simulink model "FacundoADProject2017a"  (R2017a)
settings: Solver=VariableStepAuto  StartTime=0.0  StopTime=5930  RelTol=1e-3
libraries: simulink x4, vrlib x3
settings Model: Creator=izacu  LastModifiedBy=izacu
settings DataIOCC: ReturnWorkspaceOutputs=on
settings DebuggingCC: UnconnectedInputMsg=none  UnconnectedOutputMsg=none  UnconnectedLineMsg=none  SFMachineParentedDataDiag=error
settings ModelReferenceCC: EnableRefExpFcnMdlSchedulingChecks=off
settings SFSimCC: SimUseLocalCustomCode=on
settings RTWCC: RTWUseLocalCustomCode=on

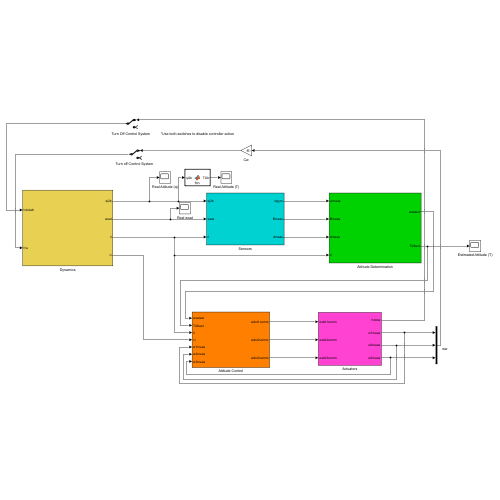
[thumbnail: Simulink's stored preview of the top-level diagram]
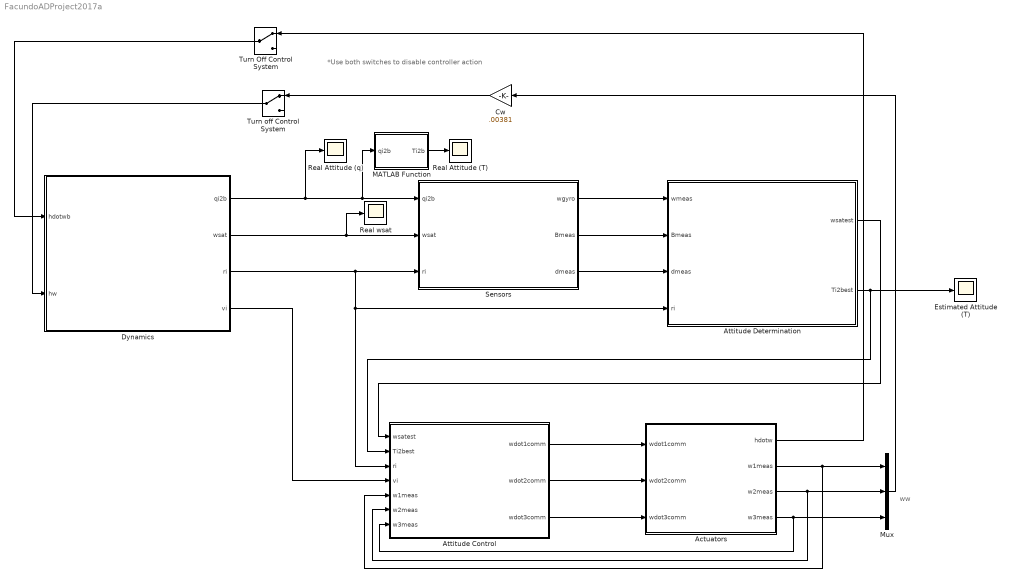
== system FacundoADProject2017a ==
  note: *Use both switches to disable controller action
  note: ww
  Actuators : Subsystem
  Attitude Control : Subsystem
  Attitude Determination : Subsystem
  Cw : Gain  Gain=.00381
  Dynamics : Subsystem
  Estimated Attitude (T) : Scope
  MATLAB Function : MATLAB Function  TreatAsAtomicUnit=on
  Mux : Mux  Inputs=3
  Real Attitude (T) : Scope
  Real Attitude (q) : Scope
  Real wsat : Scope
  Sensors : Subsystem
  Turn Off Control System : ManualSwitch
  Turn off Control System : ManualSwitch
  wires:
  Actuators/2(w1meas) -> Attitude Control/5(w1meas), Mux/1
  Actuators/3(w2meas) -> Attitude Control/6(w2meas), Mux/2
  Actuators/4(w3meas) -> Attitude Control/7(w3meas), Mux/3
  Dynamics/1(qi2b) -> Real Attitude (q)/1, MATLAB Function/1(qi2b), Sensors/1(qi2b)
  Sensors/1(wgyro) -> Attitude Determination/1(wmeas)
  Sensors/2(Bmeas) -> Attitude Determination/2(Bmeas)
  Sensors/3(dmeas) -> Attitude Determination/3(dmeas)
  Dynamics/3(ri) -> Attitude Control/3(ri), Attitude Determination/4(ri), Sensors/3(ri)
  Dynamics/2(wsat) -> Real wsat/1, Sensors/2(wsat)
  Attitude Control/1(wdot1comm) -> Actuators/1(wdot1comm)
  Attitude Control/2(wdot2comm) -> Actuators/2(wdot2comm)
  Attitude Control/3(wdot3comm) -> Actuators/3(wdot3comm)
  Dynamics/4(vi) -> Attitude Control/4(vi)
  Attitude Determination/1(wsatest) -> Attitude Control/1(wsatest)
  Attitude Determination/2(Ti2best) -> Attitude Control/2(Ti2best), Estimated Attitude (T)/1
  Mux/1 -> Cw/1
  MATLAB Function/1(Ti2b) -> Real Attitude (T)/1
  Turn off Control System/1 -> Dynamics/2(hw)
  Cw/1 -> Turn off Control System/1
  Turn Off Control System/1 -> Dynamics/1(hdotwb)
  Actuators/1(hdotw) -> Turn Off Control System/1

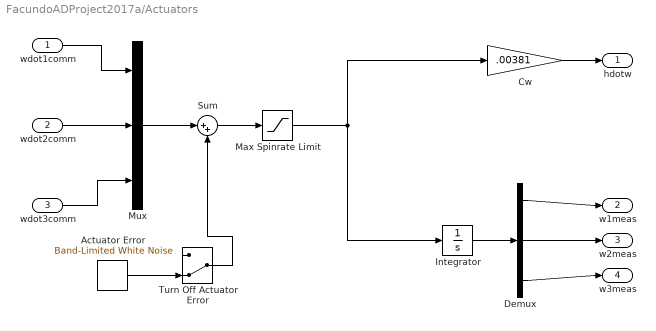
== system FacundoADProject2017a/Actuators ==
  wdot1comm : Inport
  wdot2comm : Inport  Port=2
  wdot3comm : Inport  Port=3
  Actuator Error : simulink/Sources/Band-Limited White Noise  Cov=2 * [1;1;1]  Ts=0.1  seed=[23341]
  Cw : Gain  Gain=.00381
  Demux : Demux  Outputs=3
  Integrator : Integrator  InitialCondition=[0;0;0]
  Max Spinrate Limit : Saturate  UpperLimit=262*[1;1;1]  LowerLimit=-262*[1;1;1]
  Mux : Mux  Inputs=3
  Sum : Sum  Inputs=|++
  Turn Off Actuator Error : ManualSwitch  CurrentSetting=0
  hdotw : Outport
  w1meas : Outport  Port=2
  w2meas : Outport  Port=3
  w3meas : Outport  Port=4
  wires:
  wdot1comm/1 -> Mux/1
  wdot2comm/1 -> Mux/2
  wdot3comm/1 -> Mux/3
  Mux/1 -> Sum/1
  Sum/1 -> Max Spinrate Limit/1
  Integrator/1 -> Demux/1
  Demux/1 -> w1meas/1
  Demux/2 -> w2meas/1
  Demux/3 -> w3meas/1
  Cw/1 -> hdotw/1
  Actuator Error/1 -> Turn Off Actuator Error/2
  Turn Off Actuator Error/1 -> Sum/2
  Max Spinrate Limit/1 -> Cw/1, Integrator/1

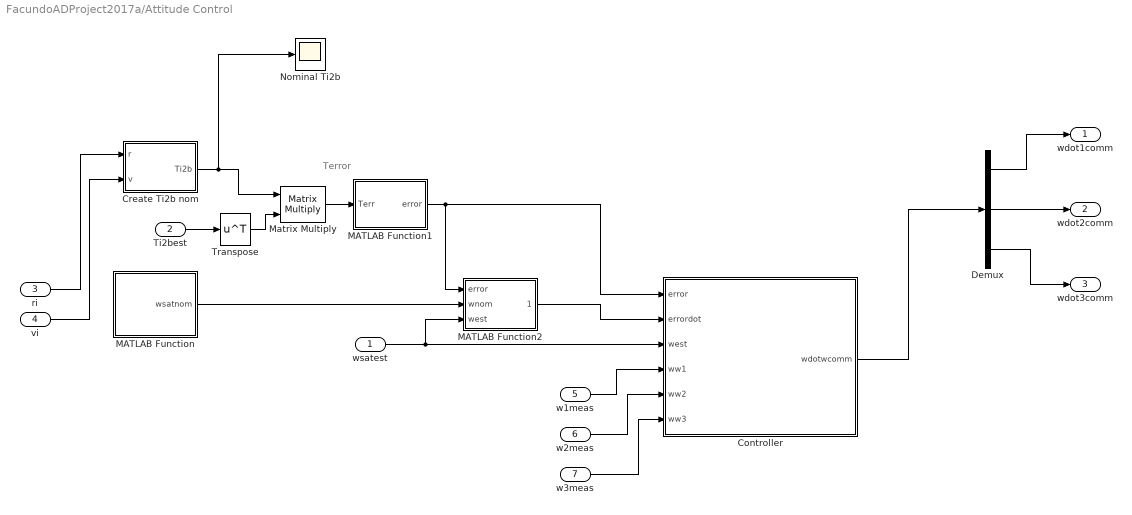
== system FacundoADProject2017a/Attitude Control ==
  note: Terror
  wsatest : Inport
  Ti2best : Inport  Port=2
  ri : Inport  Port=3
  vi : Inport  Port=4
  w1meas : Inport  Port=5
  w2meas : Inport  Port=6
  w3meas : Inport  Port=7
  Controller : MATLAB Function  TreatAsAtomicUnit=on
  Create Ti2b nom : MATLAB Function  TreatAsAtomicUnit=on
  Demux : Demux  Outputs=3
  MATLAB Function : MATLAB Function  TreatAsAtomicUnit=on
  MATLAB Function1 : MATLAB Function  TreatAsAtomicUnit=on
  MATLAB Function2 : MATLAB Function  TreatAsAtomicUnit=on
  Matrix Multiply : Product  Multiplication=Matrix(*)
  Nominal Ti2b : Scope
  Transpose : Math  Operator=transpose  SaturateOnIntegerOverflow=on
  wdot1comm : Outport
  wdot2comm : Outport  Port=2
  wdot3comm : Outport  Port=3
  wires:
  Demux/1 -> wdot1comm/1
  Demux/2 -> wdot2comm/1
  Demux/3 -> wdot3comm/1
  ri/1 -> Create Ti2b nom/1(r)
  vi/1 -> Create Ti2b nom/2(v)
  Create Ti2b nom/1(Ti2b) -> Nominal Ti2b/1, Matrix Multiply/1
  Matrix Multiply/1 -> MATLAB Function1/1(Terr)
  MATLAB Function1/1(error) -> Controller/1(error), MATLAB Function2/1(error)
  MATLAB Function/1(wsatnom) -> MATLAB Function2/2(wnom)
  wsatest/1 -> Controller/3(west), MATLAB Function2/3(west)
  Controller/1(wdotwcomm) -> Demux/1
  w1meas/1 -> Controller/4(ww1)
  w2meas/1 -> Controller/5(ww2)
  w3meas/1 -> Controller/6(ww3)
  MATLAB Function2/1(errordot) -> Controller/2(errordot)
  Ti2best/1 -> Transpose/1
  Transpose/1 -> Matrix Multiply/2

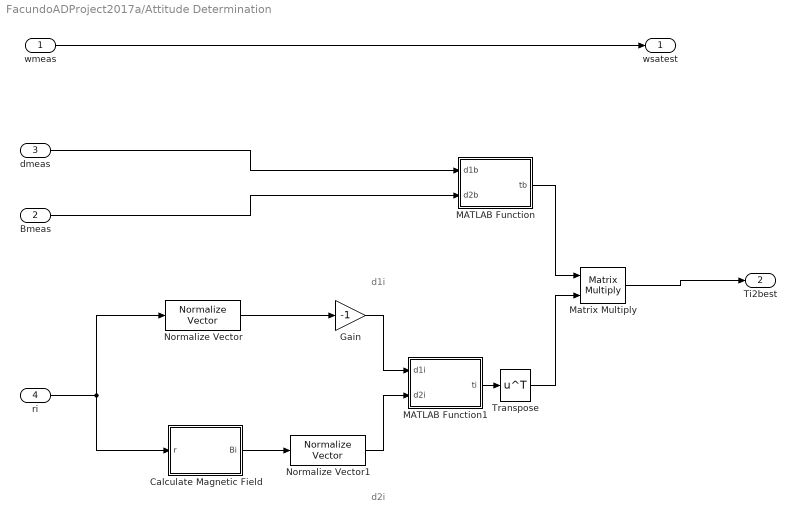
== system FacundoADProject2017a/Attitude Determination ==
  note: d2i
  note: d1i
  wmeas : Inport
  Bmeas : Inport  Port=2
  dmeas : Inport  Port=3
  ri : Inport  Port=4
  Calculate Magnetic Field : MATLAB Function  TreatAsAtomicUnit=on
  Gain : Gain  Gain=-1
  MATLAB Function : MATLAB Function  TreatAsAtomicUnit=on
  MATLAB Function1 : MATLAB Function  TreatAsAtomicUnit=on
  Matrix Multiply : Product  Multiplication=Matrix(*)
  Normalize Vector : vrlib/Utilities/Normalize Vector  maxzero=0
  Normalize Vector1 : vrlib/Utilities/Normalize Vector  maxzero=0
  Transpose : Math  Operator=transpose  SaturateOnIntegerOverflow=on
  wsatest : Outport
  Ti2best : Outport  Port=2
  wires:
  wmeas/1 -> wsatest/1
  ri/1 -> Normalize Vector/1, Calculate Magnetic Field/1(r)
  Calculate Magnetic Field/1(Bi) -> Normalize Vector1/1
  Normalize Vector/1 -> Gain/1
  dmeas/1 -> MATLAB Function/1(d1b)
  Bmeas/1 -> MATLAB Function/2(d2b)
  Gain/1 -> MATLAB Function1/1(d1i)
  Normalize Vector1/1 -> MATLAB Function1/2(d2i)
  MATLAB Function1/1(ti) -> Transpose/1
  MATLAB Function/1(tb) -> Matrix Multiply/1
  Transpose/1 -> Matrix Multiply/2
  Matrix Multiply/1 -> Ti2best/1

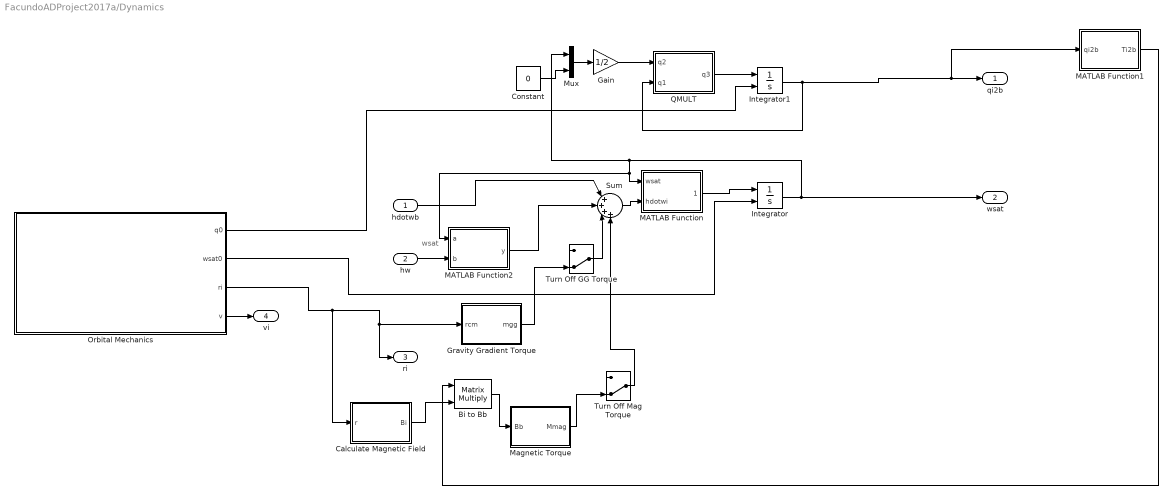
== system FacundoADProject2017a/Dynamics ==
  note: wsat
  hdotwb : Inport
  hw : Inport  Port=2
  Bi to Bb : Product  Multiplication=Matrix(*)
  Calculate Magnetic Field : MATLAB Function  TreatAsAtomicUnit=on
  Constant : Constant  Value=0
  Gain : Gain  Gain=1/2
  Gravity Gradient Torque : MATLAB Function  TreatAsAtomicUnit=on
  Integrator : Integrator  InitialConditionSource=external
  Integrator1 : Integrator  InitialConditionSource=external
  MATLAB Function : MATLAB Function  TreatAsAtomicUnit=on
  MATLAB Function1 : MATLAB Function  TreatAsAtomicUnit=on
  MATLAB Function2 : MATLAB Function  TreatAsAtomicUnit=on
  Magnetic Torque : MATLAB Function  TreatAsAtomicUnit=on
  Mux : Mux  Inputs=2
  Orbital Mechanics : Subsystem
  QMULT : MATLAB Function  TreatAsAtomicUnit=on
  Sum : Sum  Inputs=|++++
  Turn Off GG Torque : ManualSwitch  CurrentSetting=0
  Turn Off Mag Torque : ManualSwitch  CurrentSetting=0
  qi2b : Outport
  wsat : Outport  Port=2
  ri : Outport  Port=3
  vi : Outport  Port=4
  wires:
  hw/1 -> MATLAB Function2/2(b)
  hdotwb/1 -> Sum/1
  Sum/1 -> MATLAB Function/2(hdotwi)
  MATLAB Function/1(wdotsat) -> Integrator/1
  Integrator/1 -> wsat/1, Mux/1, MATLAB Function2/1(a), MATLAB Function/1(wsat)
  Orbital Mechanics/3(ri) -> Gravity Gradient Torque/1(rcm), ri/1, Calculate Magnetic Field/1(r)
  Orbital Mechanics/4(v) -> vi/1
  Orbital Mechanics/2(wsat0) -> Integrator/2
  Integrator1/1 -> QMULT/2(q1), MATLAB Function1/1(qi2b), qi2b/1
  QMULT/1(q3) -> Integrator1/1
  Mux/1 -> Gain/1
  Constant/1 -> Mux/2
  Orbital Mechanics/1(q0) -> Integrator1/2
  Gain/1 -> QMULT/1(q2)
  Calculate Magnetic Field/1(Bi) -> Bi to Bb/2
  MATLAB Function1/1(Ti2b) -> Bi to Bb/1
  Bi to Bb/1 -> Magnetic Torque/1(Bb)
  Magnetic Torque/1(Mmag) -> Turn Off Mag Torque/2
  Turn Off Mag Torque/1 -> Sum/4
  Gravity Gradient Torque/1(mgg) -> Turn Off GG Torque/2
  Turn Off GG Torque/1 -> Sum/3
  MATLAB Function2/1(y) -> Sum/2

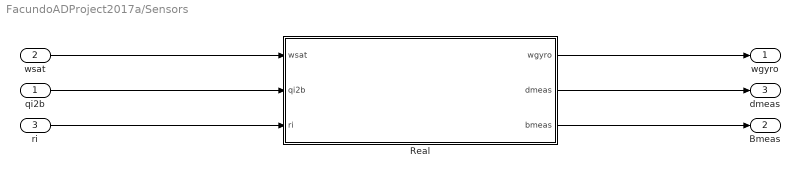
== system FacundoADProject2017a/Sensors ==
  qi2b : Inport
  wsat : Inport  Port=2
  ri : Inport  Port=3
  Real : Subsystem
  wgyro : Outport
  Bmeas : Outport  Port=2
  dmeas : Outport  Port=3
  wires:
  wsat/1 -> Real/1(wsat)
  qi2b/1 -> Real/2(qi2b)
  ri/1 -> Real/3(ri)
  Real/1(wgyro) -> wgyro/1
  Real/2(dmeas) -> dmeas/1
  Real/3(bmeas) -> Bmeas/1

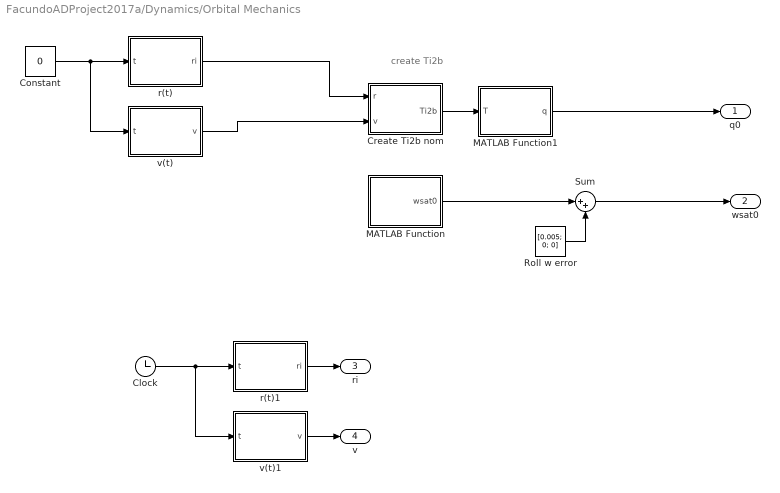
== system FacundoADProject2017a/Dynamics/Orbital Mechanics ==
  note: create Ti2b
  Clock : Clock
  Constant : Constant  Value=0
  Create Ti2b nom : MATLAB Function  TreatAsAtomicUnit=on
  MATLAB Function : MATLAB Function  TreatAsAtomicUnit=on
  MATLAB Function1 : MATLAB Function  TreatAsAtomicUnit=on
  Roll w error : Constant  Value=[0.005; 0; 0]
  Sum : Sum  Inputs=|++
  r(t) : MATLAB Function  TreatAsAtomicUnit=on
  r(t)1 : MATLAB Function  TreatAsAtomicUnit=on
  v(t) : MATLAB Function  TreatAsAtomicUnit=on
  v(t)1 : MATLAB Function  TreatAsAtomicUnit=on
  q0 : Outport
  wsat0 : Outport  Port=2
  ri : Outport  Port=3
  v : Outport  Port=4
  wires:
  Constant/1 -> v(t)/1(t), r(t)/1(t)
  v(t)/1(v) -> Create Ti2b nom/2(v)
  r(t)/1(ri) -> Create Ti2b nom/1(r)
  Roll w error/1 -> Sum/2
  MATLAB Function/1(wsat0) -> Sum/1
  Sum/1 -> wsat0/1
  Create Ti2b nom/1(Ti2b) -> MATLAB Function1/1(T)
  MATLAB Function1/1(q) -> q0/1
  Clock/1 -> v(t)1/1(t), r(t)1/1(t)
  r(t)1/1(ri) -> ri/1
  v(t)1/1(v) -> v/1

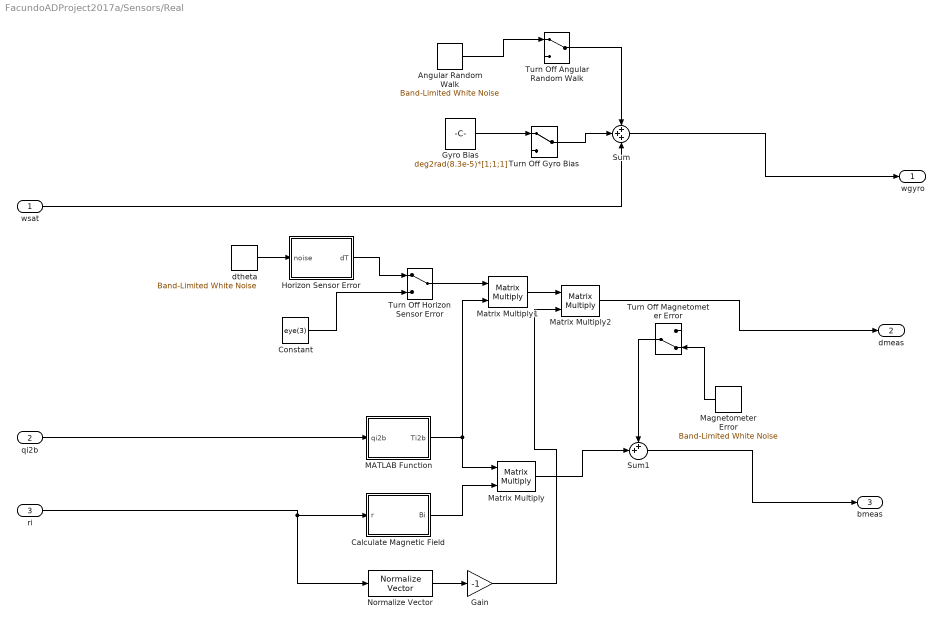
== system FacundoADProject2017a/Sensors/Real ==
  wsat : Inport
  qi2b : Inport  Port=2
  ri : Inport  Port=3
  Angular Random Walk : simulink/Sources/Band-Limited White Noise  Cov=5.29e-13 * [1; 1; 1]  Ts=0.1  seed=[23340]
  Calculate Magnetic Field : MATLAB Function  TreatAsAtomicUnit=on
  Constant : Constant  Value=eye(3)
  Gain : Gain  Gain=-1
  Gyro Bias : Constant  Value=deg2rad(8.3e-5)*[1;1;1]
  Horizon Sensor Error : MATLAB Function  TreatAsAtomicUnit=on
  MATLAB Function : MATLAB Function  TreatAsAtomicUnit=on
  Magnetometer Error : simulink/Sources/Band-Limited White Noise  Cov=[16e-40] * [1;1;1]  Ts=0.1  seed=[73341]
  Matrix Multiply : Product  Multiplication=Matrix(*)
  Matrix Multiply1 : Product  Multiplication=Matrix(*)
  Matrix Multiply2 : Product  Multiplication=Matrix(*)
  Normalize Vector : vrlib/Utilities/Normalize Vector  maxzero=0
  Sum : Sum  Inputs=+++
  Sum1 : Sum  Inputs=++|
  Turn Off Angular Random Walk : ManualSwitch
  Turn Off Gyro Bias : ManualSwitch
  Turn Off Horizon Sensor Error : ManualSwitch
  Turn Off Magnetometer Error : ManualSwitch  CurrentSetting=0
  dtheta : simulink/Sources/Band-Limited White Noise  Cov=deg2rad(0.02)*[1;1;1]  Ts=0.1  seed=[23342]
  wgyro : Outport
  dmeas : Outport  Port=2
  bmeas : Outport  Port=3
  wires:
  Matrix Multiply/1 -> Sum1/2
  Matrix Multiply2/1 -> dmeas/1
  ri/1 -> Normalize Vector/1, Calculate Magnetic Field/1(r)
  Matrix Multiply1/1 -> Matrix Multiply2/1
  MATLAB Function/1(Ti2b) -> Matrix Multiply1/2, Matrix Multiply/1
  Calculate Magnetic Field/1(Bi) -> Matrix Multiply/2
  Gain/1 -> Matrix Multiply2/2
  qi2b/1 -> MATLAB Function/1(qi2b)
  Normalize Vector/1 -> Gain/1
  Sum1/1 -> bmeas/1
  wsat/1 -> Sum/3
  Sum/1 -> wgyro/1
  dtheta/1 -> Horizon Sensor Error/1(noise)
  Magnetometer Error/1 -> Turn Off Magnetometer Error/2
  Turn Off Magnetometer Error/1 -> Sum1/1
  Constant/1 -> Turn Off Horizon Sensor Error/2
  Turn Off Horizon Sensor Error/1 -> Matrix Multiply1/1
  Horizon Sensor Error/1(dT) -> Turn Off Horizon Sensor Error/1
  Gyro Bias/1 -> Turn Off Gyro Bias/1
  Turn Off Gyro Bias/1 -> Sum/2
  Angular Random Walk/1 -> Turn Off Angular Random Walk/1
  Turn Off Angular Random Walk/1 -> Sum/1

== matlab function FacundoADProject2017a/Dynamics/MATLAB Function ==
  data: wsat input; wdotsat output; hdotwi input
function wdotsat = fcn(wsat,hdotwi)

J = [17.53 0 0;
     0 11.97 0;
     0 0 11.97];

wdotsat = inv(J) * (cross(-wsat,(J*wsat)) - hdotwi); %#ok<MINV> 
end

== matlab function FacundoADProject2017a/Dynamics/Orbital Mechanics/r(t) ==
  data: t input; ri output
function ri = fcn(t)

p = 7.078e6; % m (7078km)
mu = 3.986e14;
w = sqrt(mu / (p^3));

ri = (p/sqrt(2)) * [-cos(w*t); sqrt(2)*sin(w*t); cos(w*t)];

== matlab function FacundoADProject2017a/Dynamics/Orbital Mechanics/v(t) ==
  data: t input; v output
function v = fcn(t)

p = 6600;
mu = 398600;
w = sqrt(mu / (p^3));

v = (w*p/sqrt(2)) * [sin(w*t); sqrt(2)*cos(w*t); -sin(w*t)];

== matlab function FacundoADProject2017a/Sensors/Real/MATLAB Function ==
  data: qi2b input; Ti2b output
function Ti2b = fcn(qi2b)

I = eye(3);
qs = qi2b(4);
qv = [qi2b(1:3)];

Ti2b = I - 2*qs*skewsym(qv) + 2*(skewsym(qv))^2;

end

function skewed = skewsym(v)
skewed = [0 -v(3) v(2);
          v(3) 0 -v(1);
          -v(2) v(1) 0];
end

== matlab function FacundoADProject2017a/Sensors/Real/Calculate Magnetic Field ==
  data: r input; Bi output
function Bi = fcn(r)

Re = 6378; % km
B0 = 3.12e-5; % T

nz = -r./norm(r);
ny = cross(nz, [0; 0; 1]) ./ norm(cross(nz, [0; 0; 1]));
nx = cross(ny,nz);
Ti2n = [nx'; ny'; nz'];

lat = acos(r(3)/norm(r));

Bn = (B0*(Re/norm(r))^3) * [cos(lat); 0; -2*sin(lat)];

Bi = Ti2n*Bn;

== matlab function FacundoADProject2017a/Sensors/Real/Horizon Sensor Error ==
  data: noise input; dT output
function dT = fcn(noise)

angle = norm(noise);

axis = noise/norm(noise);

dT = eye(3) - sin(angle)*skewsym(axis) + (1 - cos(angle)) * skewsym(axis)^2;

end

function skewed = skewsym(v)
skewed = [0 -v(3) v(2);
          v(3) 0 -v(1);
          -v(2) v(1) 0];
end

== matlab function FacundoADProject2017a/Attitude Determination/Calculate Magnetic Field ==
  data: r input; Bi output
function Bi = fcn(r)

Re = 6378; % km
B0 = 3.12e-5; % T

nz = -r./norm(r);
ny = cross(nz, [0; 0; 1]) ./ norm(cross(nz, [0; 0; 1]));
nx = cross(ny,nz);
Ti2n = [nx'; ny'; nz'];

lat = acos(r(3)/norm(r));

Bn = (B0*(Re/norm(r))^3) * [cos(lat); 0; -2*sin(lat)];

Bi = Ti2n*Bn;

== matlab function FacundoADProject2017a/Attitude Determination/MATLAB Function ==
  data: d1b input; tb output; d2b input
function tb = fcn(d1b,d2b)

tbx = d1b;

tbz = cross(d1b,d2b) / norm(cross(d1b,d2b));

tby = cross(tbz,tbx);

tb = [tbx tby tbz];

end

== matlab function FacundoADProject2017a/Attitude Determination/MATLAB Function1 ==
  data: d1i input; ti output; d2i input
function ti = fcn(d1i,d2i)

tix = d1i;

tiz = cross(d1i,d2i) / norm(cross(d1i,d2i));

tiy = cross(tiz,tix);

ti = [tix tiy tiz];

== matlab function FacundoADProject2017a/Dynamics/QMULT ==
  data: q2 input; q3 output; q1 input
function q3 = qmult(q2,q1)

q3 = [q2(4).*q1(1:3) + q1(4).*q2(1:3) - cross(q2(1:3),q1(1:3));
    q2(4)*q1(4) - dot(q2(1:3),q1(1:3))];

end

== matlab function FacundoADProject2017a/Dynamics/Orbital Mechanics/Create Ti2b nom ==
  data: r input; Ti2b output; v input
function Ti2b = fcn(r,v)

xib = -r / norm(r);
yib = v / norm(v);
zib = cross(xib,yib);

Ti2b = [xib'; yib'; zib'];

== matlab function FacundoADProject2017a/Dynamics/Orbital Mechanics/MATLAB Function ==
  data: wsat0 output
function wsat0= fcn()
mu = 3.986e14;
rho = 6.6e6;
wmag = sqrt(mu / rho^3);

wsat0 = wmag .* [0;0;1];

== matlab function FacundoADProject2017a/Dynamics/Orbital Mechanics/MATLAB Function1 ==
  data: T input; q output
function q = T2q(T)

q = zeros(4,1);

q(4) = sqrt(.25*(1 + T(1,1) + T(2,2) + T(3,3)));

q = (1/(4*q(4))) .* [T(2,3) - T(3,2); T(3,1) + T(1,3); T(1,2) + T(2,1); 4 * q(4)^2 ];

end

== matlab function FacundoADProject2017a/Attitude Control/Create Ti2b nom ==
  data: r input; Ti2b output; v input
function Ti2b = fcn(r,v)

xib = -r / norm(r);
yib = v / norm(v);
zib = cross(xib,yib);

Ti2b = [xib'; yib'; zib'];

== matlab function FacundoADProject2017a/Attitude Control/MATLAB Function ==
  data: wsatnom output
function wsatnom = fcn()
mu = 398600.0;
rho = 6600;
wmag = sqrt(mu / rho^3);



wsatnom = wmag .* [0;0;1];

== matlab function FacundoADProject2017a/Attitude Control/MATLAB Function1 ==
  data: Terr input; error output
function error = fcn(Terr)

error = -0.5 * [Terr(3,2) - Terr(2,3); 
                Terr(1,3) - Terr(3,1); 
                Terr(2,1) - Terr(1,2)];

== matlab function FacundoADProject2017a/Attitude Control/MATLAB Function2 ==
  data: error input; wnom input; errordot output; west input
function errordot = fcn(error,wnom,west)

errordot = -skewsym(wnom)*error + (wnom - west);

end

function skewed = skewsym(v)
skewed = [0 -v(3) v(2);
          v(3) 0 -v(1);
          -v(2) v(1) 0];
end

== matlab function FacundoADProject2017a/Attitude Control/Controller ==
  data: error input; wdotwcomm output; errordot input; west input; ww1 input; ww2 input; ww3 input
function wdotwcomm = fcn(error,errordot,west,ww1,ww2,ww3)
Jsat = [17.53 0 0; 0 11.97 0; 0 0 11.97];
Kd = -0.08*eye(3);
Kp = -0.05*eye(3);
Cw = .00381;
% calculate control torque (first two terms of next line)
wdotwcomm = (Jsat*Kp ./ Cw) * error + (Jsat*Kd ./ Cw) * errordot - cross(west, [ww1; ww2; ww3]);
% bypass actuators to provide torque to dynamics block

== matlab function FacundoADProject2017a/Dynamics/Orbital Mechanics/r(t)1 ==
  data: t input; ri output
function ri = fcn(t)

p = 7.078e6;
mu = 3.986e14;
w = sqrt(mu / (p^3));

ri = (p/sqrt(2)) * [-cos(w*t); sqrt(2)*sin(w*t); cos(w*t)];

== matlab function FacundoADProject2017a/Dynamics/Orbital Mechanics/v(t)1 ==
  data: t input; v output
function v = fcn(t)

p = 7.078e6;
mu = 3.986e14;
w = sqrt(mu / (p^3));

v = (w*p/sqrt(2)) * [sin(w*t); sqrt(2)*cos(w*t); -sin(w*t)];

== matlab function FacundoADProject2017a/Dynamics/Gravity Gradient Torque ==
  data: rcm input; mgg output
function mgg = fcn(rcm)
J = [17.53 0 0;
     0 11.97 0;
     0 0 11.97];
mu = 3.986e14;
worb = sqrt(mu / norm(rcm)^3);
d = -rcm / norm(rcm);

mgg = cross(3*(worb^2)*d, J*d);

== matlab function FacundoADProject2017a/Dynamics/MATLAB Function1 ==
  data: qi2b input; Ti2b output
function Ti2b = fcn(qi2b)

I = eye(3);
qs = qi2b(4);
qv = [qi2b(1:3)];

Ti2b = I - 2*qs*skewsym(qv) + 2*(skewsym(qv))^2;

end

function skewed = skewsym(v)
skewed = [0 -v(3) v(2);
          v(3) 0 -v(1);
          -v(2) v(1) 0];
end

== matlab function FacundoADProject2017a/Dynamics/MATLAB Function2 ==
  data: a input; y output; b input
function y = crossprod(a,b)

y = cross(a,b);

== matlab function FacundoADProject2017a/MATLAB Function ==
  data: qi2b input; Ti2b output
function Ti2b = fcn(qi2b)

I = eye(3);
qs = qi2b(4);
qv = [qi2b(1:3)];

Ti2b = I - 2*qs*skewsym(qv) + 2*(skewsym(qv))^2;

end

function skewed = skewsym(v)
skewed = [0 -v(3) v(2);
          v(3) 0 -v(1);
          -v(2) v(1) 0];
end

== matlab function FacundoADProject2017a/Dynamics/Calculate Magnetic Field ==
  data: r input; Bi output
function Bi = fcn(r)

Re = 6378; % km
B0 = 3.12e-5; % T

nz = -r./norm(r);
ny = cross(nz, [0; 0; 1]) ./ norm(cross(nz, [0; 0; 1]));
nx = cross(ny,nz);
Ti2n = [nx'; ny'; nz'];

lat = acos(r(3)/norm(r));

Bn = (B0*(Re/norm(r))^3) * [cos(lat); 0; -2*sin(lat)];

Bi = Ti2n*Bn;

== matlab function FacundoADProject2017a/Dynamics/Magnetic Torque ==
  data: Bb input; Mmag output
function Mmag = fcn(Bb)
mu = [.896; 0; 0]; % Nm / Tesla
Mmag = cross(mu, Bb);
